simulink model "simulink_pidcontroller"  (R2014b)
settings: Solver=ode45  StartTime=0.0  StopTime=t_sim  FixedStep=0.1  MaxStep=0.01  RelTol=1e-6
values from neighbouring files (symbols this model uses):
  D = 0.1143    [main.m]
  I = 0.72939    [main.m]
  i_a0 = 0    [main.m]
  J_m = 0.01    [main.m]
  K_E = 1    [main.m]
  K_M = 1    [main.m]
  L_a = 1    [main.m]
  M_L = 0    [main.m]
  N = 899.2487    [main.m]
  P = 5.3286    [main.m]
  R_a = 10    [main.m]
  theta_0 = 0    [main.m]
  theta_r = pi/2    (= 1.57079632679)    [main.m]
  w_m0 = 0    [main.m]
libraries: simulink x1
settings Model: Creator=rende_000  LastModifiedBy=rende_000

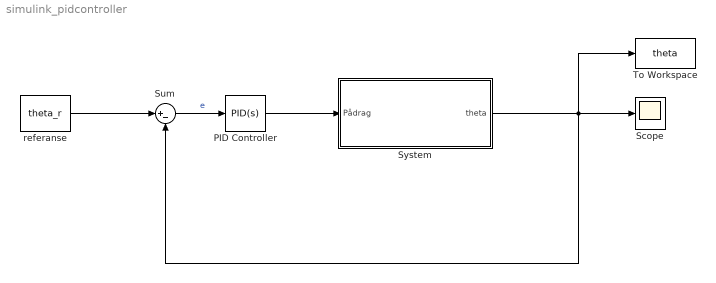
== system simulink_pidcontroller ==
  PID Controller : simulink/Continuous/PID Controller  Controller=PID  TimeDomain=Continuous-time  SampleTime=-1  IntegratorMethod=Forward Euler  FilterMethod=Forward Euler  Form=Ideal  P=P  I=I  D=D  N=N  InitialConditionSource=internal  InitialConditionForIntegrator=0  InitialConditionForFilter=0  ExternalReset=none  LimitOutput=off  UpperSaturationLimit=inf  LowerSaturationLimit=-inf  LinearizeAsGain=on  AntiWindupMode=none  Kb=1  TrackingMode=off  Kt=1  PParamMin=[]  PParamMax=[]  IParamMin=[]  IParamMax=[]  DParamMin=[]  DParamMax=[]  NParamMin=[]  NParamMax=[]  KbParamMin=[]  KbParamMax=[]  KtParamMin=[]  KtParamMax=[]  POutMin=[]  POutMax=[]  IOutMin=[]  IOutMax=[]  DOutMin=[]  DOutMax=[]  NOutMin=[]  NOutMax=[]  KbOutMin=[]  KbOutMax=[]  KtOutMin=[]  KtOutMax=[]  IntegratorOutMin=[]  IntegratorOutMax=[]  FilterOutMin=[]  FilterOutMax=[]  SumOutMin=[]  SumOutMax=[]  SumI1OutMin=[]  SumI1OutMax=[]  SumI2OutMin=[]  SumI2OutMax=[]  SumI3OutMin=[]  SumI3OutMax=[]  SumDOutMin=[]  SumDOutMax=[]  SaturationOutMin=[]  SaturationOutMax=[]  IntegratorContinuousStateAttributes=''  IntegratorStateMustResolveToSignalObject=off  IntegratorRTWStateStorageClass=Auto  FilterContinuousStateAttributes=''  FilterStateMustResolveToSignalObject=off  FilterRTWStateStorageClass=Auto  DifferentiatorICPrevScaledInput=0  DifferentiatorOutMin=[]  DifferentiatorOutMax=[]  UseFilter=on
  Scope : Scope
  Sum : Sum  Inputs=|+-
  System : Subsystem
  To Workspace : ToWorkspace  VariableName=theta  SaveFormat=Timeseries  SampleTime=-1
  referanse : Constant  Value=theta_r
  wires:
  System/1(theta) -> To Workspace/1, Scope/1, Sum/2
  Sum/1 -> PID Controller/1  "e"
  PID Controller/1 -> System/1(Pådrag)
  referanse/1 -> Sum/1

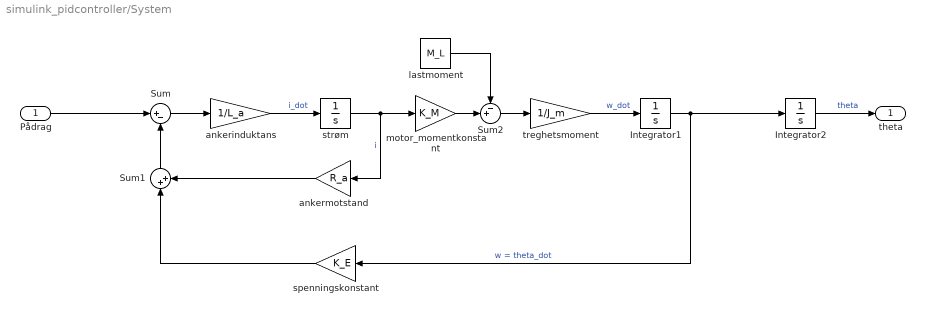
== system simulink_pidcontroller/System ==
  Pådrag : Inport
  Integrator1 : Integrator  InitialCondition=w_m0
  Integrator2 : Integrator  InitialCondition=theta_0
  Sum : Sum  Inputs=|+-
  Sum1 : Sum  Inputs=|++
  Sum2 : Sum  Inputs=-+|
  ankerinduktans : Gain  Gain=1/L_a
  ankermotstand : Gain  Gain=R_a
  lastmoment : Constant  Value=M_L
  motor_momentkonstant : Gain  Gain=K_M
  spenningskonstant : Gain  Gain=K_E
  strøm : Integrator  InitialCondition=i_a0
  treghetsmoment : Gain  Gain=1/J_m
  theta : Outport
  wires:
  ankerinduktans/1 -> strøm/1  "i_dot"
  Sum/1 -> ankerinduktans/1
  strøm/1 -> motor_momentkonstant/1, ankermotstand/1  "i"
  Sum2/1 -> treghetsmoment/1
  lastmoment/1 -> Sum2/1
  Integrator1/1 -> spenningskonstant/1, Integrator2/1  "w = theta_dot"
  Sum1/1 -> Sum/2
  ankermotstand/1 -> Sum1/2
  spenningskonstant/1 -> Sum1/1
  Integrator2/1 -> theta/1  "theta"
  motor_momentkonstant/1 -> Sum2/2
  Pådrag/1 -> Sum/1
  treghetsmoment/1 -> Integrator1/1  "w_dot"
